simulink library "PC_Simulator_Lib"  (Simulink 8.2)
settings: Solver=ode45  StartTime=0.0  StopTime=10.0  RelTol=1e-3
values from neighbouring files (symbols this model uses):
  data = [r1 r2 r3 r4 L1 L2 L3 L4]    [strasse_Bedatung_HNI_ITI.m]
  distSameLane = 60    [InitialisationsEnv.m]
  eng_speed = [0 60 120 180 240 300 360 420 480 540 600 660 ... (101 elements, 1x101)]    [engine_table.mat]    (also in motor_parameter_calc.m = omega)
  Heading_init = 0    [Start.m]
  inertiaLateral = 25*(radiusWheel)^2    (= 4.129024)    [Start.m]
  laneWidth = 3.6    [InitialisationsEnv.m]    (also in strasse_Bedatung_HNI_ITI.m)
  omega_engine = [0.000000 150.000000 500.000000 1000.000000 1500.000000 2000.000000 2500.000000 3000.000000 3500.000000 4000.000000 4500.000000 5000.000000 5500.000000 6000.000000]    [friction_tables.m]
  omega_max = 6000    [engine_table.mat]    (also in motor_parameter_calc.m)
  omega_wheel = [0 20 40 60 80 100 122 143.7 164]    [friction_tables.m]
  para_Fellow_8_Points = ADAS.Fellow_8_Points    [ADAS_parameters.m]
  position_start_x = [x1 x2 x3 x4 x5 x6 x7]    [strasse_Bedatung_HNI_ITI.m]
  position_start_y = [y1 y2 y3 y4 y5 y6 y7]    [strasse_Bedatung_HNI_ITI.m]
  rad3rdLine = 57.2    [InitialisationsEnv.m]    (also in strasse_Bedatung_HNI_ITI.m)
  radiusWheel = 16*2.54/100    (= 0.4064)    [Start.m]
  s_values = [S1 S2 S3 S4 S5 S6 S7]    [strasse_Bedatung_HNI_ITI.m]
  segmentLimits = [segment1EndThirdLine                   segment2EndThirdLine                   segment3EndThirdLine                   segment4EndThirdLine                   segment5EndThirdLine                   segment6EndThirdLine                   segment7EndThirdLine                   segment8EndThirdLine                   ]    [InitialisationsEnv.m]    (also in strasse_Bedatung_HNI_ITI.m)
  setPosT = [-1.8 -5.4 -1.8 -5.4 -1.8 -5.4 -1.8 -5.4 -1.8 -5.4]    [InitialisationsEnv.m]
  torque = [297.089227105 300.997600937 304.800343044 308.497453426 312.088932082 315.574779014 318.95499422 322.229577701 325.398529457 328.461849487 331.419537793 334.271594373 ... (101 elements, 1x101)]    [engine_table.mat]    (also in motor_parameter_calc.m = g)
  Torque_lost = [0.000000 -8.777780 -15.000000 -26.800000 -29.600000 -32.700000 -35.900000 -39.300000 -42.800000 -46.500000 -50.300000 -54.300000 -58.500000 -62.800000 ]*0.6    [friction_tables.m]
  Torque_lost_wheel = [0.8 0.8 0.75 0.7 0.4 0.3 0.2 0.07 0.07]*0.2    [friction_tables.m]
  X_init = 0    [Start.m]
  Y_init = 1.8    [Start.m]
  Z_init = 0    [Start.m]
undefined symbols (not defined in the file or in its folder): Acc_Pedal, ADAS, Brake_Pedal, Joystick, Newton, Para, Raphson, Standard_Devices, Steering_Wheel_Angle, UDP_Protocol
libraries: simulink x43, rtwinlib x7, dspnetwork x2, simulink_extras x1, vrlib x1
(part 11 of 13)

== system PC_Simulator_Lib/Vehicle dynamics/Vertical_Dyn./suspention_System/Rear_Right_Suspention/vertical_dynamics_tire ==
  note: U
  note: F0
  note: z1
  Force_Suspention : Inport
  Vertical_Displacement_Z0_Road : Inport  Port=2
  intial_force_form_mass : Inport  Port=3
  1/Mu : Gain  Gain=1/Para.VD.wheel_Mass.v
  Add1 : Sum  Inputs=++-
  Add2 : Sum  Inputs=+-
  Gain : Gain  Gain=Para.VD.Tire_Stifness.v
  Gain2 : Gain  Gain=Para.VD.Tire_Damping_Constant.v
  Integrator : Integrator
  Integrator1 : Integrator
  Relational Operator : RelationalOperator  Operator=>  OutDataTypeStr=boolean  ZeroCross=off
  Saturation : Saturate  UpperLimit=Para.VD.Tire_intial_length.v-Para.VD.Tire_Lower_limit.v  LowerLimit=Para.VD.Tire_intial_length.v-Para.VD.Tire_Upper_limit.v
  Subtract2 : Sum  Inputs=+-
  Subtract3 : Sum  Inputs=+-
  Sum : Sum  Inputs=|++
  Switch : Switch
  Transfer Fcn : TransferFcn  Numerator=[1 0]  Denominator=[0.001 1]
  Transfer Fcn1 : TransferFcn  Numerator=[1 0]  Denominator=[0.001 1]
  Vertical_Displacement_Z1_Wheel : Outport
  Vertical_Velocity_Z1_Wheel : Outport  Port=2
  wires:
  Transfer Fcn1/1 -> Vertical_Velocity_Z1_Wheel/1
  Add1/1 -> 1/Mu/1
  1/Mu/1 -> Integrator/1
  Integrator/1 -> Integrator1/1, Subtract3/2
  Integrator1/1 -> Subtract2/2, Switch/3
  Subtract3/1 -> Gain2/1
  Gain2/1 -> Add1/2
  Saturation/1 -> Gain/1, Relational Operator/2, Add2/2
  Subtract2/1 -> Saturation/1, Relational Operator/1
  Transfer Fcn/1 -> Subtract3/1
  Vertical_Displacement_Z0_Road/1 -> Add2/1, Subtract2/1, Transfer Fcn/1
  Force_Suspention/1 -> Add1/3
  Gain/1 -> Sum/2
  Sum/1 -> Add1/1
  intial_force_form_mass/1 -> Sum/1
  Add2/1 -> Switch/1
  Relational Operator/1 -> Switch/2
  Switch/1 -> Transfer Fcn1/1, Vertical_Displacement_Z1_Wheel/1

== system PC_Simulator_Lib/Vehicle dynamics/Vertical_Dyn./suspention_System/Rear_left_Suspention/vertical_dynamics_tire ==
  note: U
  note: F0
  note: z1
  Force_Suspention : Inport
  Vertical_Displacement_Z0_Road : Inport  Port=2
  intial_force_form_mass : Inport  Port=3
  1/Mu : Gain  Gain=1/Para.VD.wheel_Mass.v
  Add1 : Sum  Inputs=++-
  Add2 : Sum  Inputs=+-
  Gain : Gain  Gain=Para.VD.Tire_Stifness.v
  Gain2 : Gain  Gain=Para.VD.Tire_Damping_Constant.v
  Integrator : Integrator
  Integrator1 : Integrator
  Relational Operator : RelationalOperator  Operator=>  OutDataTypeStr=boolean  ZeroCross=off
  Saturation : Saturate  UpperLimit=Para.VD.Tire_intial_length.v-Para.VD.Tire_Lower_limit.v  LowerLimit=Para.VD.Tire_intial_length.v-Para.VD.Tire_Upper_limit.v
  Subtract2 : Sum  Inputs=+-
  Subtract3 : Sum  Inputs=+-
  Sum : Sum  Inputs=|++
  Switch : Switch
  Transfer Fcn : TransferFcn  Numerator=[1 0]  Denominator=[0.001 1]
  Transfer Fcn1 : TransferFcn  Numerator=[1 0]  Denominator=[0.001 1]
  Vertical_Displacement_Z1_Wheel : Outport
  Vertical_Velocity_Z1_Wheel : Outport  Port=2
  wires:
  Transfer Fcn1/1 -> Vertical_Velocity_Z1_Wheel/1
  Add1/1 -> 1/Mu/1
  1/Mu/1 -> Integrator/1
  Integrator/1 -> Integrator1/1, Subtract3/2
  Integrator1/1 -> Subtract2/2, Switch/3
  Subtract3/1 -> Gain2/1
  Gain2/1 -> Add1/2
  Saturation/1 -> Gain/1, Relational Operator/2, Add2/2
  Subtract2/1 -> Saturation/1, Relational Operator/1
  Transfer Fcn/1 -> Subtract3/1
  Vertical_Displacement_Z0_Road/1 -> Add2/1, Subtract2/1, Transfer Fcn/1
  Force_Suspention/1 -> Add1/3
  Gain/1 -> Sum/2
  Sum/1 -> Add1/1
  intial_force_form_mass/1 -> Sum/1
  Add2/1 -> Switch/1
  Relational Operator/1 -> Switch/2
  Switch/1 -> Transfer Fcn1/1, Vertical_Displacement_Z1_Wheel/1

== system PC_Simulator_Lib/Vehicle dynamics/Vertical_Dyn./suspention_System/front_left_Suspention/vertical_dynamics_tire ==
  note: U
  note: F0
  note: z1
  Force_Suspention : Inport
  Vertical_Displacement_Z0_Road : Inport  Port=2
  intial_force_form_mass : Inport  Port=3
  1/Mu : Gain  Gain=1/Para.VD.wheel_Mass.v
  Add1 : Sum  Inputs=++-
  Add2 : Sum  Inputs=+-
  Gain : Gain  Gain=Para.VD.Tire_Stifness.v
  Gain2 : Gain  Gain=Para.VD.Tire_Damping_Constant.v
  Integrator : Integrator
  Integrator1 : Integrator
  Relational Operator : RelationalOperator  Operator=>  OutDataTypeStr=boolean  ZeroCross=off
  Saturation : Saturate  UpperLimit=Para.VD.Tire_intial_length.v-Para.VD.Tire_Lower_limit.v  LowerLimit=Para.VD.Tire_intial_length.v-Para.VD.Tire_Upper_limit.v
  Subtract2 : Sum  Inputs=+-
  Subtract3 : Sum  Inputs=+-
  Sum : Sum  Inputs=|++
  Switch : Switch
  Transfer Fcn : TransferFcn  Numerator=[1 0]  Denominator=[0.001 1]
  Transfer Fcn1 : TransferFcn  Numerator=[1 0]  Denominator=[0.001 1]
  Vertical_Displacement_Z1_Wheel : Outport
  Vertical_Velocity_Z1_Wheel : Outport  Port=2
  wires:
  Transfer Fcn1/1 -> Vertical_Velocity_Z1_Wheel/1
  Add1/1 -> 1/Mu/1
  1/Mu/1 -> Integrator/1
  Integrator/1 -> Integrator1/1, Subtract3/2
  Integrator1/1 -> Subtract2/2, Switch/3
  Subtract3/1 -> Gain2/1
  Gain2/1 -> Add1/2
  Saturation/1 -> Gain/1, Relational Operator/2, Add2/2
  Subtract2/1 -> Saturation/1, Relational Operator/1
  Transfer Fcn/1 -> Subtract3/1
  Vertical_Displacement_Z0_Road/1 -> Add2/1, Subtract2/1, Transfer Fcn/1
  Force_Suspention/1 -> Add1/3
  Gain/1 -> Sum/2
  Sum/1 -> Add1/1
  intial_force_form_mass/1 -> Sum/1
  Add2/1 -> Switch/1
  Relational Operator/1 -> Switch/2
  Switch/1 -> Transfer Fcn1/1, Vertical_Displacement_Z1_Wheel/1

== system PC_Simulator_Lib/Vehicle dynamics/Vertical_Dyn./suspention_System/front_right_Suspention/vertical_dynamics_tire ==
  note: U
  note: F0
  note: z1
  Force_Suspention : Inport
  Vertical_Displacement_Z0_Road : Inport  Port=2
  intial_force_form_mass : Inport  Port=3
  1/Mu : Gain  Gain=1/Para.VD.wheel_Mass.v
  Add1 : Sum  Inputs=++-
  Add2 : Sum  Inputs=+-
  Gain : Gain  Gain=Para.VD.Tire_Stifness.v
  Gain2 : Gain  Gain=Para.VD.Tire_Damping_Constant.v
  Integrator : Integrator
  Integrator1 : Integrator
  Relational Operator : RelationalOperator  Operator=>  OutDataTypeStr=boolean  ZeroCross=off
  Saturation : Saturate  UpperLimit=Para.VD.Tire_intial_length.v-Para.VD.Tire_Lower_limit.v  LowerLimit=Para.VD.Tire_intial_length.v-Para.VD.Tire_Upper_limit.v
  Subtract2 : Sum  Inputs=+-
  Subtract3 : Sum  Inputs=+-
  Sum : Sum  Inputs=|++
  Switch : Switch
  Transfer Fcn : TransferFcn  Numerator=[1 0]  Denominator=[0.001 1]
  Transfer Fcn1 : TransferFcn  Numerator=[1 0]  Denominator=[0.001 1]
  Vertical_Displacement_Z1_Wheel : Outport
  Vertical_Velocity_Z1_Wheel : Outport  Port=2
  wires:
  Transfer Fcn1/1 -> Vertical_Velocity_Z1_Wheel/1
  Add1/1 -> 1/Mu/1
  1/Mu/1 -> Integrator/1
  Integrator/1 -> Integrator1/1, Subtract3/2
  Integrator1/1 -> Subtract2/2, Switch/3
  Subtract3/1 -> Gain2/1
  Gain2/1 -> Add1/2
  Saturation/1 -> Gain/1, Relational Operator/2, Add2/2
  Subtract2/1 -> Saturation/1, Relational Operator/1
  Transfer Fcn/1 -> Subtract3/1
  Vertical_Displacement_Z0_Road/1 -> Add2/1, Subtract2/1, Transfer Fcn/1
  Force_Suspention/1 -> Add1/3
  Gain/1 -> Sum/2
  Sum/1 -> Add1/1
  intial_force_form_mass/1 -> Sum/1
  Add2/1 -> Switch/1
  Relational Operator/1 -> Switch/2
  Switch/1 -> Transfer Fcn1/1, Vertical_Displacement_Z1_Wheel/1

== system PC_Simulator_Lib/ADAS/Decision_Making_ADAS/Trajectory_calculatin_and_distance_control_and output_maping/Calculate_Desired_Trajectory/applying_Desired_T_Gradually/Triggered Subsystem ==
  In1 : Inport
  Trigger : TriggerPort  TriggerType=either
  Out1 : Outport
  wires:
  In1/1 -> Out1/1

== system PC_Simulator_Lib/ADAS/Decision_Making_ADAS/Trajectory_calculatin_and_distance_control_and output_maping/Distance_Control/Distance controller/Control_law ==
  Distance_desired[m] : Inport
  Distance_acctual[m] : Inport  Port=2
  V_realtive[m|s] : Inport  Port=3
  V_Vehicle[m|s] : Inport  Port=4
  V_Desired_max[m|s] : Inport  Port=5
  V_Desired_min[m|s] : Inport  Port=6
  Enable : EnablePort  StatesWhenEnabling=reset
  Add : Sum  Inputs=+++
  Add1 : Sum
  Add2 : Sum
  Ground : Ground
  Integrator : Integrator
  Kb : Gain  Gain=0.02
  Ki : Gain  Gain=0.001
  Kp : Gain  Gain=0.2
  Saturation Dynamic : simulink/Discontinuities/Saturation Dynamic  OutMin=[]  OutMax=[]  OutDataTypeStr=Inherit: Same as second input  OutDataType=fixdt(1, 16)  OutScaling=2^-10  DoSatur=off
  Subtract1 : Sum  Inputs=-+
  Subtract2 : Sum  Inputs=-+
  Terminator : Terminator
  V_Desired_Following[m|s] : Outport
  wires:
  Distance_desired[m]/1 -> Subtract1/1
  Distance_acctual[m]/1 -> Subtract1/2
  Subtract1/1 -> Kp/1, Ki/1
  Integrator/1 -> Terminator/1
  Kp/1 -> Add/2
  Add1/1 -> Integrator/1
  Ki/1 -> Add1/1
  Kb/1 -> Add1/2
  Saturation Dynamic/1 -> V_Desired_Following[m|s]/1, Subtract2/2
  V_Desired_max[m|s]/1 -> Saturation Dynamic/1
  V_Desired_min[m|s]/1 -> Saturation Dynamic/3
  Add/1 -> Saturation Dynamic/2, Subtract2/1
  V_Vehicle[m|s]/1 -> Add2/2
  V_realtive[m|s]/1 -> Add2/1
  Add2/1 -> Add/1
  Subtract2/1 -> Kb/1
  Ground/1 -> Add/3

== system PC_Simulator_Lib/ADAS/Decision_Making_ADAS/Trajectory_calculatin_and_distance_control_and output_maping/Distance_Control/Distance controller/Enable_Distance_Controller ==
  S_Start_Braking[m] : Inport
  Distance_2_Felow_Vehicle[m] : Inport  Port=2
  V_realtive[m|s] : Inport  Port=3
  V_Vehicle[m|s] : Inport  Port=4
  V_User_Set_Speed[m|s] : Inport  Port=5
  Add2 : Sum
  Gain : Gain  Gain=1.2
  Logical Operator : Logic  AllPortsSameDT=off  OutDataTypeStr=boolean
  Relational Operator : RelationalOperator  Operator=>  OutDataTypeStr=boolean
  Relational Operator1 : RelationalOperator  Operator=<  OutDataTypeStr=boolean
  Relational Operator2 : RelationalOperator  Operator=>  OutDataTypeStr=boolean
  S-R Flip-Flop : simulink_extras/Flip Flops/S-R Flip-Flop  initial_condition=0
  Terminator : Terminator
  Enable_Distance_Controller : Outport
  wires:
  Distance_2_Felow_Vehicle[m]/1 -> Relational Operator1/2, Relational Operator/2
  S_Start_Braking[m]/1 -> Gain/1, Relational Operator/1
  Relational Operator/1 -> S-R Flip-Flop/1
  S-R Flip-Flop/2 -> Terminator/1
  Relational Operator1/1 -> Logical Operator/1
  V_realtive[m|s]/1 -> Add2/1
  V_Vehicle[m|s]/1 -> Add2/2
  Add2/1 -> Relational Operator2/1
  V_User_Set_Speed[m|s]/1 -> Relational Operator2/2
  Logical Operator/1 -> S-R Flip-Flop/2
  Relational Operator2/1 -> Logical Operator/2
  S-R Flip-Flop/1 -> Enable_Distance_Controller/1
  Gain/1 -> Relational Operator1/1

== system PC_Simulator_Lib/ADAS/Execution_ADAS/Longitudinal_Controller/Acceleration_Control/Tractive_Force_Required_determination/Force_of_Aerodynamics ==
  Vx_CoG[m|s] : Inport
  Gain : Gain  Gain=Para.VD.Air_Risistance_Coefficient.v
  Math Function : Math  Operator=square  SaturateOnIntegerOverflow=on
  Product2 : Product  RndMeth=Zero
  Sign : Signum
  Force_of_aerodynamics_in_X : Outport
  wires:
  Vx_CoG[m|s]/1 -> Math Function/1, Sign/1
  Sign/1 -> Product2/2
  Gain/1 -> Product2/1
  Product2/1 -> Force_of_aerodynamics_in_X/1
  Math Function/1 -> Gain/1

== system PC_Simulator_Lib/ADAS/Execution_ADAS/Longitudinal_Controller/Acceleration_Control/Tractive_Force_Required_determination/Friction_FL ==
  omega_radPs : Inport
  Lookup Table : Lookup_n-D  NumberOfTableDimensions=1  BreakpointsForDimension1=omega_wheel  BeginIndexSearchUsingPreviousIndexResult=on  Table=Torque_lost_wheel  InputSameDT=on
  Product : Product  RndMeth=Zero
  Torque_friction : Outport
  wires:
  omega_radPs/1 -> Product/2, Lookup Table/1
  Product/1 -> Torque_friction/1
  Lookup Table/1 -> Product/1

== system PC_Simulator_Lib/ADAS/Execution_ADAS/Longitudinal_Controller/Acceleration_Control/Tractive_Force_Required_determination/Friction_FR ==
  omega_radPs : Inport
  Lookup Table : Lookup_n-D  NumberOfTableDimensions=1  BreakpointsForDimension1=omega_wheel  BeginIndexSearchUsingPreviousIndexResult=on  Table=Torque_lost_wheel  InputSameDT=on
  Product : Product  RndMeth=Zero
  Torque_friction : Outport
  wires:
  Lookup Table/1 -> Product/1
  Product/1 -> Torque_friction/1
  omega_radPs/1 -> Lookup Table/1, Product/2

== system PC_Simulator_Lib/ADAS/Execution_ADAS/Longitudinal_Controller/Acceleration_Control/Tractive_Force_Required_determination/Friction_RL ==
  omega_radPs : Inport
  Lookup Table : Lookup_n-D  NumberOfTableDimensions=1  BreakpointsForDimension1=omega_wheel  BeginIndexSearchUsingPreviousIndexResult=on  Table=Torque_lost_wheel  InputSameDT=on
  Product : Product  RndMeth=Zero
  Torque_friction : Outport
  wires:
  omega_radPs/1 -> Product/2, Lookup Table/1
  Product/1 -> Torque_friction/1
  Lookup Table/1 -> Product/1

== system PC_Simulator_Lib/ADAS/Execution_ADAS/Longitudinal_Controller/Acceleration_Control/Tractive_Force_Required_determination/Friction_RR ==
  omega_radPs : Inport
  Lookup Table : Lookup_n-D  NumberOfTableDimensions=1  BreakpointsForDimension1=omega_wheel  BeginIndexSearchUsingPreviousIndexResult=on  Table=Torque_lost_wheel  InputSameDT=on
  Product : Product  RndMeth=Zero
  Torque_friction : Outport
  wires:
  Lookup Table/1 -> Product/1
  Product/1 -> Torque_friction/1
  omega_radPs/1 -> Lookup Table/1, Product/2

== system PC_Simulator_Lib/ADAS/Sensors_ADAS/Front_Long_Range_Radar_Sensor/First_STage_Coordinate_Transformation/Radar_Triangles_Transformation_From_Local2Global/Pitch_angle_offset ==
  Constant : Constant  Value=0.02
  Constant1 : Constant  Value=7*pi/180
  Digital Clock : DigitalClock  SampleTime=0.001
  Gain : Gain  Gain=1000
  Gain1 : Gain  Gain=atan(1/250)*3
  Math Function : Math  Operator=rem  SaturateOnIntegerOverflow=on
  Subtract : Sum  Inputs=+-
  Delta_pitch_angle[rad] : Outport
  Round_done[bool] : Outport  Port=2
  wires:
  Digital Clock/1 -> Math Function/1
  Gain1/1 -> Subtract/1
  Constant/1 -> Math Function/2
  Gain/1 -> Gain1/1, Round_done[bool]/1
  Math Function/1 -> Gain/1
  Subtract/1 -> Delta_pitch_angle[rad]/1
  Constant1/1 -> Subtract/2

== system PC_Simulator_Lib/ADAS/Sensors_ADAS/Front_Long_Range_Radar_Sensor/First_STage_Coordinate_Transformation/Radar_Triangles_Transformation_From_Local2Global/Subsystem ==
  Transformation_Local2Global : Inport
  Position_of_Origine_Local_coord[m] : Inport  Port=2
  Positon_Local[m] : Inport  Port=3
  Add1 : Sum
  Product1 : Product  Multiplication=Matrix(*)
  Position_Global[m] : Outport
  wires:
  Positon_Local[m]/1 -> Product1/2
  Transformation_Local2Global/1 -> Product1/1
  Position_of_Origine_Local_coord[m]/1 -> Add1/2
  Add1/1 -> Position_Global[m]/1
  Product1/1 -> Add1/1

== system PC_Simulator_Lib/ADAS/Sensors_ADAS/Front_Long_Range_Radar_Sensor/First_STage_Coordinate_Transformation/Radar_Triangles_Transformation_From_Local2Global/Subsystem1 ==
  Transformation_Local2Global : Inport
  Position_of_Origine_Local_coord[m] : Inport  Port=2
  Positon_Local[m] : Inport  Port=3
  Add1 : Sum
  Product1 : Product  Multiplication=Matrix(*)
  Position_Global[m] : Outport
  wires:
  Product1/1 -> Add1/1
  Add1/1 -> Position_Global[m]/1
  Position_of_Origine_Local_coord[m]/1 -> Add1/2
  Transformation_Local2Global/1 -> Product1/1
  Positon_Local[m]/1 -> Product1/2

== system PC_Simulator_Lib/ADAS/Sensors_ADAS/Front_Long_Range_Radar_Sensor/First_STage_Coordinate_Transformation/Radar_Triangles_Transformation_From_Local2Global/Subsystem2 ==
  Transformation_Local2Global : Inport
  Position_of_Origine_Local_coord[m] : Inport  Port=2
  Positon_Local[m] : Inport  Port=3
  Add1 : Sum
  Product1 : Product  Multiplication=Matrix(*)
  Position_Global[m] : Outport
  wires:
  Positon_Local[m]/1 -> Product1/2
  Transformation_Local2Global/1 -> Product1/1
  Position_of_Origine_Local_coord[m]/1 -> Add1/2
  Add1/1 -> Position_Global[m]/1
  Product1/1 -> Add1/1

== system PC_Simulator_Lib/ADAS/Sensors_ADAS/Front_Long_Range_Radar_Sensor/First_STage_Coordinate_Transformation/Radar_Triangles_Transformation_From_Local2Global/Subsystem3 ==
  Transformation_Local2Global : Inport
  Position_of_Origine_Local_coord[m] : Inport  Port=2
  Positon_Local[m] : Inport  Port=3
  Add1 : Sum
  Product1 : Product  Multiplication=Matrix(*)
  Position_Global[m] : Outport
  wires:
  Product1/1 -> Add1/1
  Add1/1 -> Position_Global[m]/1
  Position_of_Origine_Local_coord[m]/1 -> Add1/2
  Transformation_Local2Global/1 -> Product1/1
  Positon_Local[m]/1 -> Product1/2

== system PC_Simulator_Lib/ADAS/Sensors_ADAS/Front_Long_Range_Radar_Sensor/First_STage_Coordinate_Transformation/Radar_Triangles_Transformation_From_Local2Global/Subsystem4 ==
  Transformation_Local2Global : Inport
  Position_of_Origine_Local_coord[m] : Inport  Port=2
  Positon_Local[m] : Inport  Port=3
  Add1 : Sum
  Product1 : Product  Multiplication=Matrix(*)
  Position_Global[m] : Outport
  wires:
  Positon_Local[m]/1 -> Product1/2
  Transformation_Local2Global/1 -> Product1/1
  Position_of_Origine_Local_coord[m]/1 -> Add1/2
  Add1/1 -> Position_Global[m]/1
  Product1/1 -> Add1/1

== system PC_Simulator_Lib/ADAS/Sensors_ADAS/Front_Long_Range_Radar_Sensor/First_STage_Coordinate_Transformation/Radar_Triangles_Transformation_From_Local2Global/Subsystem5 ==
  Transformation_Local2Global : Inport
  Position_of_Origine_Local_coord[m] : Inport  Port=2
  Positon_Local[m] : Inport  Port=3
  Add1 : Sum
  Product1 : Product  Multiplication=Matrix(*)
  Position_Global[m] : Outport
  wires:
  Product1/1 -> Add1/1
  Add1/1 -> Position_Global[m]/1
  Position_of_Origine_Local_coord[m]/1 -> Add1/2
  Transformation_Local2Global/1 -> Product1/1
  Positon_Local[m]/1 -> Product1/2

== system PC_Simulator_Lib/ADAS/Sensors_ADAS/Front_Long_Range_Radar_Sensor/First_STage_Coordinate_Transformation/Radar_Triangles_Transformation_From_Local2Global/Subsystem6 ==
  Transformation_Local2Global : Inport
  Position_of_Origine_Local_coord[m] : Inport  Port=2
  Positon_Local[m] : Inport  Port=3
  Add1 : Sum
  Product1 : Product  Multiplication=Matrix(*)
  Position_Global[m] : Outport
  wires:
  Positon_Local[m]/1 -> Product1/2
  Transformation_Local2Global/1 -> Product1/1
  Position_of_Origine_Local_coord[m]/1 -> Add1/2
  Add1/1 -> Position_Global[m]/1
  Product1/1 -> Add1/1

== system PC_Simulator_Lib/ADAS/Sensors_ADAS/Front_Long_Range_Radar_Sensor/First_STage_Coordinate_Transformation/Radar_Triangles_Transformation_From_Local2Global/Subsystem7 ==
  Transformation_Local2Global : Inport
  Position_of_Origine_Local_coord[m] : Inport  Port=2
  Positon_Local[m] : Inport  Port=3
  Add1 : Sum
  Product1 : Product  Multiplication=Matrix(*)
  Position_Global[m] : Outport
  wires:
  Product1/1 -> Add1/1
  Add1/1 -> Position_Global[m]/1
  Position_of_Origine_Local_coord[m]/1 -> Add1/2
  Transformation_Local2Global/1 -> Product1/1
  Positon_Local[m]/1 -> Product1/2

== system PC_Simulator_Lib/ADAS/Sensors_ADAS/Front_Mid_Range_Radar_Sensor/First_STage_Coordinate_Transformation/Radar_Triangles_Transformation_From_Local2Global/Pitch_angle_offset ==
  Constant : Constant  Value=0.02
  Constant1 : Constant  Value=7*pi/180
  Digital Clock : DigitalClock  SampleTime=0.001
  Gain : Gain  Gain=1000
  Gain1 : Gain  Gain=atan(1/250)*3
  Math Function : Math  Operator=rem  SaturateOnIntegerOverflow=on
  Subtract : Sum  Inputs=+-
  Delta_pitch_angle[rad] : Outport
  Round_done[bool] : Outport  Port=2
  wires:
  Digital Clock/1 -> Math Function/1
  Gain1/1 -> Subtract/1
  Constant/1 -> Math Function/2
  Gain/1 -> Gain1/1, Round_done[bool]/1
  Math Function/1 -> Gain/1
  Subtract/1 -> Delta_pitch_angle[rad]/1
  Constant1/1 -> Subtract/2

== system PC_Simulator_Lib/ADAS/Sensors_ADAS/Front_Mid_Range_Radar_Sensor/First_STage_Coordinate_Transformation/Radar_Triangles_Transformation_From_Local2Global/Subsystem ==
  Transformation_Local2Global : Inport
  Position_of_Origine_Local_coord[m] : Inport  Port=2
  Positon_Local[m] : Inport  Port=3
  Add1 : Sum
  Product1 : Product  Multiplication=Matrix(*)
  Position_Global[m] : Outport
  wires:
  Positon_Local[m]/1 -> Product1/2
  Transformation_Local2Global/1 -> Product1/1
  Position_of_Origine_Local_coord[m]/1 -> Add1/2
  Add1/1 -> Position_Global[m]/1
  Product1/1 -> Add1/1

== system PC_Simulator_Lib/ADAS/Sensors_ADAS/Front_Mid_Range_Radar_Sensor/First_STage_Coordinate_Transformation/Radar_Triangles_Transformation_From_Local2Global/Subsystem1 ==
  Transformation_Local2Global : Inport
  Position_of_Origine_Local_coord[m] : Inport  Port=2
  Positon_Local[m] : Inport  Port=3
  Add1 : Sum
  Product1 : Product  Multiplication=Matrix(*)
  Position_Global[m] : Outport
  wires:
  Product1/1 -> Add1/1
  Add1/1 -> Position_Global[m]/1
  Position_of_Origine_Local_coord[m]/1 -> Add1/2
  Transformation_Local2Global/1 -> Product1/1
  Positon_Local[m]/1 -> Product1/2

== system PC_Simulator_Lib/ADAS/Sensors_ADAS/Front_Mid_Range_Radar_Sensor/First_STage_Coordinate_Transformation/Radar_Triangles_Transformation_From_Local2Global/Subsystem2 ==
  Transformation_Local2Global : Inport
  Position_of_Origine_Local_coord[m] : Inport  Port=2
  Positon_Local[m] : Inport  Port=3
  Add1 : Sum
  Product1 : Product  Multiplication=Matrix(*)
  Position_Global[m] : Outport
  wires:
  Positon_Local[m]/1 -> Product1/2
  Transformation_Local2Global/1 -> Product1/1
  Position_of_Origine_Local_coord[m]/1 -> Add1/2
  Add1/1 -> Position_Global[m]/1
  Product1/1 -> Add1/1

== system PC_Simulator_Lib/ADAS/Sensors_ADAS/Front_Mid_Range_Radar_Sensor/First_STage_Coordinate_Transformation/Radar_Triangles_Transformation_From_Local2Global/Subsystem3 ==
  Transformation_Local2Global : Inport
  Position_of_Origine_Local_coord[m] : Inport  Port=2
  Positon_Local[m] : Inport  Port=3
  Add1 : Sum
  Product1 : Product  Multiplication=Matrix(*)
  Position_Global[m] : Outport
  wires:
  Product1/1 -> Add1/1
  Add1/1 -> Position_Global[m]/1
  Position_of_Origine_Local_coord[m]/1 -> Add1/2
  Transformation_Local2Global/1 -> Product1/1
  Positon_Local[m]/1 -> Product1/2

== system PC_Simulator_Lib/ADAS/Sensors_ADAS/Front_Mid_Range_Radar_Sensor/First_STage_Coordinate_Transformation/Radar_Triangles_Transformation_From_Local2Global/Subsystem4 ==
  Transformation_Local2Global : Inport
  Position_of_Origine_Local_coord[m] : Inport  Port=2
  Positon_Local[m] : Inport  Port=3
  Add1 : Sum
  Product1 : Product  Multiplication=Matrix(*)
  Position_Global[m] : Outport
  wires:
  Positon_Local[m]/1 -> Product1/2
  Transformation_Local2Global/1 -> Product1/1
  Position_of_Origine_Local_coord[m]/1 -> Add1/2
  Add1/1 -> Position_Global[m]/1
  Product1/1 -> Add1/1

== system PC_Simulator_Lib/ADAS/Sensors_ADAS/Front_Mid_Range_Radar_Sensor/First_STage_Coordinate_Transformation/Radar_Triangles_Transformation_From_Local2Global/Subsystem5 ==
  Transformation_Local2Global : Inport
  Position_of_Origine_Local_coord[m] : Inport  Port=2
  Positon_Local[m] : Inport  Port=3
  Add1 : Sum
  Product1 : Product  Multiplication=Matrix(*)
  Position_Global[m] : Outport
  wires:
  Product1/1 -> Add1/1
  Add1/1 -> Position_Global[m]/1
  Position_of_Origine_Local_coord[m]/1 -> Add1/2
  Transformation_Local2Global/1 -> Product1/1
  Positon_Local[m]/1 -> Product1/2

== system PC_Simulator_Lib/ADAS/Sensors_ADAS/Front_Mid_Range_Radar_Sensor/First_STage_Coordinate_Transformation/Radar_Triangles_Transformation_From_Local2Global/Subsystem6 ==
  Transformation_Local2Global : Inport
  Position_of_Origine_Local_coord[m] : Inport  Port=2
  Positon_Local[m] : Inport  Port=3
  Add1 : Sum
  Product1 : Product  Multiplication=Matrix(*)
  Position_Global[m] : Outport
  wires:
  Positon_Local[m]/1 -> Product1/2
  Transformation_Local2Global/1 -> Product1/1
  Position_of_Origine_Local_coord[m]/1 -> Add1/2
  Add1/1 -> Position_Global[m]/1
  Product1/1 -> Add1/1

== system PC_Simulator_Lib/ADAS/Sensors_ADAS/Front_Mid_Range_Radar_Sensor/First_STage_Coordinate_Transformation/Radar_Triangles_Transformation_From_Local2Global/Subsystem7 ==
  Transformation_Local2Global : Inport
  Position_of_Origine_Local_coord[m] : Inport  Port=2
  Positon_Local[m] : Inport  Port=3
  Add1 : Sum
  Product1 : Product  Multiplication=Matrix(*)
  Position_Global[m] : Outport
  wires:
  Product1/1 -> Add1/1
  Add1/1 -> Position_Global[m]/1
  Position_of_Origine_Local_coord[m]/1 -> Add1/2
  Transformation_Local2Global/1 -> Product1/1
  Positon_Local[m]/1 -> Product1/2

== system PC_Simulator_Lib/ADAS/Sensors_ADAS/Input_Maping/Fellows/Subsystem2/Subsystem1 ==
  In1 : Inport
  Constant9 : Constant  Value=Z_init
  Sum : Sum  Inputs=|++
  Out1 : Outport
  wires:
  Sum/1 -> Out1/1
  Constant9/1 -> Sum/2
  In1/1 -> Sum/1

== system PC_Simulator_Lib/ADAS/Sensors_ADAS/Input_Maping/Fellows/Subsystem2/Subsystem10 ==
  In1 : Inport
  Constant9 : Constant  Value=Z_init
  Sum : Sum  Inputs=|++
  Out1 : Outport
  wires:
  Sum/1 -> Out1/1
  Constant9/1 -> Sum/2
  In1/1 -> Sum/1

== system PC_Simulator_Lib/ADAS/Sensors_ADAS/Input_Maping/Fellows/Subsystem2/Subsystem2 ==
  In1 : Inport
  Constant9 : Constant  Value=Z_init
  Sum : Sum  Inputs=|++
  Out1 : Outport
  wires:
  In1/1 -> Sum/1
  Constant9/1 -> Sum/2
  Sum/1 -> Out1/1

== system PC_Simulator_Lib/ADAS/Sensors_ADAS/Input_Maping/Fellows/Subsystem2/Subsystem3 ==
  In1 : Inport
  Constant9 : Constant  Value=Z_init
  Sum : Sum  Inputs=|++
  Out1 : Outport
  wires:
  Sum/1 -> Out1/1
  Constant9/1 -> Sum/2
  In1/1 -> Sum/1

== system PC_Simulator_Lib/ADAS/Sensors_ADAS/Input_Maping/Fellows/Subsystem2/Subsystem4 ==
  In1 : Inport
  Constant9 : Constant  Value=Z_init
  Sum : Sum  Inputs=|++
  Out1 : Outport
  wires:
  In1/1 -> Sum/1
  Constant9/1 -> Sum/2
  Sum/1 -> Out1/1

== system PC_Simulator_Lib/ADAS/Sensors_ADAS/Input_Maping/Fellows/Subsystem2/Subsystem5 ==
  In1 : Inport
  Constant9 : Constant  Value=Z_init
  Sum : Sum  Inputs=|++
  Out1 : Outport
  wires:
  Sum/1 -> Out1/1
  Constant9/1 -> Sum/2
  In1/1 -> Sum/1

== system PC_Simulator_Lib/ADAS/Sensors_ADAS/Input_Maping/Fellows/Subsystem2/Subsystem6 ==
  In1 : Inport
  Constant9 : Constant  Value=Z_init
  Sum : Sum  Inputs=|++
  Out1 : Outport
  wires:
  In1/1 -> Sum/1
  Constant9/1 -> Sum/2
  Sum/1 -> Out1/1

== system PC_Simulator_Lib/ADAS/Sensors_ADAS/Input_Maping/Fellows/Subsystem2/Subsystem7 ==
  In1 : Inport
  Constant9 : Constant  Value=Z_init
  Sum : Sum  Inputs=|++
  Out1 : Outport
  wires:
  Sum/1 -> Out1/1
  Constant9/1 -> Sum/2
  In1/1 -> Sum/1

== system PC_Simulator_Lib/ADAS/Sensors_ADAS/Input_Maping/Fellows/Subsystem2/Subsystem8 ==
  In1 : Inport
  Constant9 : Constant  Value=Z_init
  Sum : Sum  Inputs=|++
  Out1 : Outport
  wires:
  In1/1 -> Sum/1
  Constant9/1 -> Sum/2
  Sum/1 -> Out1/1

== system PC_Simulator_Lib/ADAS/Sensors_ADAS/Input_Maping/Fellows/Subsystem2/Subsystem9 ==
  In1 : Inport
  Constant9 : Constant  Value=Z_init
  Sum : Sum  Inputs=|++
  Out1 : Outport
  wires:
  In1/1 -> Sum/1
  Constant9/1 -> Sum/2
  Sum/1 -> Out1/1

== system PC_Simulator_Lib/Drive_Train/4_Wheels_drive_train_and_Brake/FL/Alpha_Kappa_Selector2/Dynamik Anteil2/Subsystem3 ==
  In1 : Inport
  Abs : Abs  SaturateOnIntegerOverflow=on
  In3_Switch : Constant
  Relational Operator : RelationalOperator
  Switch : Switch  Threshold=1  SaturateOnIntegerOverflow=on
  Out1 : Outport
  wires:
  In1/1 -> Switch/1, Abs/1
  Abs/1 -> Relational Operator/1
  In3_Switch/1 -> Relational Operator/2, Switch/3
  Relational Operator/1 -> Switch/2
  Switch/1 -> Out1/1

== system PC_Simulator_Lib/Drive_Train/4_Wheels_drive_train_and_Brake/FL/Alpha_Kappa_Selector2/alpha_calc/Slip_angle_Calculation_From_Vx_and_Vy1 ==
  Vx_CoG[m|s] : Inport
  Vy_CoG[m|s] : Inport  Port=2
  Add : Sum
  Add2 : Sum
  Compare To Constant1 : simulink/Logic and Bit Operations/Compare To Constant  relop=>=  const=1  OutDataTypeStr=boolean
  Constant1 : Constant  Value=eps
  Data Type Conversion : DataTypeConversion
  Divide : Product  Inputs=*/
  Gain : Gain  Gain=180/pi
  Math Function : Math  Operator=square  SaturateOnIntegerOverflow=on
  Math Function1 : Math  Operator=square  SaturateOnIntegerOverflow=on
  Product1 : Product  Inputs=3
  Sign : Signum
  Sqrt : Sqrt  AlgorithmType=Newton-Raphson  SaturateOnIntegerOverflow=on
  Trigonometric Function1 : Trigonometry  Operator=atan
  Unary Minus1 : UnaryMinus
  Slip_Angle[deg] : Outport
  wires:
  Gain/1 -> Slip_Angle[deg]/1
  Product1/1 -> Gain/1
  Data Type Conversion/1 -> Product1/2
  Compare To Constant1/1 -> Data Type Conversion/1
  Vy_CoG[m|s]/1 -> Math Function1/1, Divide/1
  Vx_CoG[m|s]/1 -> Sign/1, Math Function/1, Add2/1
  Math Function/1 -> Add/1
  Math Function1/1 -> Add/2
  Add/1 -> Sqrt/1
  Sqrt/1 -> Compare To Constant1/1
  Divide/1 -> Trigonometric Function1/1
  Add2/1 -> Divide/2
  Constant1/1 -> Add2/2
  Trigonometric Function1/1 -> Product1/1
  Sign/1 -> Unary Minus1/1
  Unary Minus1/1 -> Product1/3

== system PC_Simulator_Lib/Drive_Train/4_Wheels_drive_train_and_Brake/FL/Alpha_Kappa_Selector2/alpha_calc/front ==
  Vy : Inport
  Vx : Inport  Port=2
  steering_angle : Inport  Port=3
  Constant : Constant  Value=0.001
  Divide : Product  Inputs=*/
  Fcn : Fcn  Expr=atan(u)
  Gain : Gain  Gain=180/pi
  Relational Operator : RelationalOperator  OutDataTypeStr=boolean
  Subsystem1 : Subsystem
  Subtract : Sum  Inputs=+-
  Switch : Switch  Threshold=1
  alpha : Outport
  wires:
  Relational Operator/1 -> Switch/2
  Constant/1 -> Switch/3, Relational Operator/2
  steering_angle/1 -> Subtract/1
  Subtract/1 -> Gain/1
  Divide/1 -> Fcn/1
  Gain/1 -> alpha/1
  Fcn/1 -> Subtract/2
  Switch/1 -> Divide/2
  Vy/1 -> Subsystem1/1(In1)
  Vx/1 -> Relational Operator/1, Switch/1
  Subsystem1/1(Out1) -> Divide/1

== system PC_Simulator_Lib/Drive_Train/4_Wheels_drive_train_and_Brake/FR/Alpha_Kappa_Selector2/Dynamik Anteil2/Subsystem3 ==
  In1 : Inport
  Abs : Abs  SaturateOnIntegerOverflow=on
  In3_Switch : Constant
  Relational Operator : RelationalOperator
  Switch : Switch  Threshold=1  SaturateOnIntegerOverflow=on
  Out1 : Outport
  wires:
  In1/1 -> Switch/1, Abs/1
  Abs/1 -> Relational Operator/1
  In3_Switch/1 -> Relational Operator/2, Switch/3
  Relational Operator/1 -> Switch/2
  Switch/1 -> Out1/1

== system PC_Simulator_Lib/Drive_Train/4_Wheels_drive_train_and_Brake/FR/Alpha_Kappa_Selector2/alpha_calc/Slip_angle_Calculation_From_Vx_and_Vy1 ==
  Vx_CoG[m|s] : Inport
  Vy_CoG[m|s] : Inport  Port=2
  Add : Sum
  Add2 : Sum
  Compare To Constant1 : simulink/Logic and Bit Operations/Compare To Constant  relop=>=  const=1  OutDataTypeStr=boolean
  Constant1 : Constant  Value=eps
  Data Type Conversion : DataTypeConversion
  Divide : Product  Inputs=*/
  Gain : Gain  Gain=180/pi
  Math Function : Math  Operator=square  SaturateOnIntegerOverflow=on
  Math Function1 : Math  Operator=square  SaturateOnIntegerOverflow=on
  Product1 : Product  Inputs=3
  Sign : Signum
  Sqrt : Sqrt  AlgorithmType=Newton-Raphson  SaturateOnIntegerOverflow=on
  Trigonometric Function1 : Trigonometry  Operator=atan
  Unary Minus1 : UnaryMinus
  Slip_Angle[deg] : Outport
  wires:
  Gain/1 -> Slip_Angle[deg]/1
  Product1/1 -> Gain/1
  Data Type Conversion/1 -> Product1/2
  Compare To Constant1/1 -> Data Type Conversion/1
  Vy_CoG[m|s]/1 -> Math Function1/1, Divide/1
  Vx_CoG[m|s]/1 -> Sign/1, Math Function/1, Add2/1
  Math Function/1 -> Add/1
  Math Function1/1 -> Add/2
  Add/1 -> Sqrt/1
  Sqrt/1 -> Compare To Constant1/1
  Divide/1 -> Trigonometric Function1/1
  Add2/1 -> Divide/2
  Constant1/1 -> Add2/2
  Trigonometric Function1/1 -> Product1/1
  Sign/1 -> Unary Minus1/1
  Unary Minus1/1 -> Product1/3

== system PC_Simulator_Lib/Drive_Train/4_Wheels_drive_train_and_Brake/FR/Alpha_Kappa_Selector2/alpha_calc/front ==
  Vy : Inport
  Vx : Inport  Port=2
  steering_angle : Inport  Port=3
  Constant : Constant  Value=0.001
  Divide : Product  Inputs=*/
  Fcn : Fcn  Expr=atan(u)
  Gain : Gain  Gain=180/pi
  Relational Operator : RelationalOperator  OutDataTypeStr=boolean
  Subsystem1 : Subsystem
  Subtract : Sum  Inputs=+-
  Switch : Switch  Threshold=1
  alpha : Outport
  wires:
  Relational Operator/1 -> Switch/2
  Constant/1 -> Switch/3, Relational Operator/2
  steering_angle/1 -> Subtract/1
  Subtract/1 -> Gain/1
  Divide/1 -> Fcn/1
  Gain/1 -> alpha/1
  Fcn/1 -> Subtract/2
  Switch/1 -> Divide/2
  Vy/1 -> Subsystem1/1(In1)
  Vx/1 -> Relational Operator/1, Switch/1
  Subsystem1/1(Out1) -> Divide/1

== system PC_Simulator_Lib/Drive_Train/4_Wheels_drive_train_and_Brake/RL/Alpha_Kappa_Selector2/Dynamik Anteil2/Subsystem3 ==
  In1 : Inport
  Abs : Abs  SaturateOnIntegerOverflow=on
  In3_Switch : Constant
  Relational Operator : RelationalOperator
  Switch : Switch  Threshold=1  SaturateOnIntegerOverflow=on
  Out1 : Outport
  wires:
  In1/1 -> Switch/1, Abs/1
  Abs/1 -> Relational Operator/1
  In3_Switch/1 -> Relational Operator/2, Switch/3
  Relational Operator/1 -> Switch/2
  Switch/1 -> Out1/1

== system PC_Simulator_Lib/Drive_Train/4_Wheels_drive_train_and_Brake/RL/Alpha_Kappa_Selector2/alpha_calc/Slip_angle_Calculation_From_Vx_and_Vy1 ==
  Vx_CoG[m|s] : Inport
  Vy_CoG[m|s] : Inport  Port=2
  Add : Sum
  Add2 : Sum
  Compare To Constant1 : simulink/Logic and Bit Operations/Compare To Constant  relop=>=  const=1  OutDataTypeStr=boolean
  Constant1 : Constant  Value=eps
  Data Type Conversion : DataTypeConversion
  Divide : Product  Inputs=*/
  Gain : Gain  Gain=180/pi
  Math Function : Math  Operator=square  SaturateOnIntegerOverflow=on
  Math Function1 : Math  Operator=square  SaturateOnIntegerOverflow=on
  Product1 : Product  Inputs=3
  Sign : Signum
  Sqrt : Sqrt  AlgorithmType=Newton-Raphson  SaturateOnIntegerOverflow=on
  Trigonometric Function1 : Trigonometry  Operator=atan
  Unary Minus1 : UnaryMinus
  Slip_Angle[deg] : Outport
  wires:
  Gain/1 -> Slip_Angle[deg]/1
  Product1/1 -> Gain/1
  Data Type Conversion/1 -> Product1/2
  Compare To Constant1/1 -> Data Type Conversion/1
  Vy_CoG[m|s]/1 -> Math Function1/1, Divide/1
  Vx_CoG[m|s]/1 -> Sign/1, Math Function/1, Add2/1
  Math Function/1 -> Add/1
  Math Function1/1 -> Add/2
  Add/1 -> Sqrt/1
  Sqrt/1 -> Compare To Constant1/1
  Divide/1 -> Trigonometric Function1/1
  Add2/1 -> Divide/2
  Constant1/1 -> Add2/2
  Trigonometric Function1/1 -> Product1/1
  Sign/1 -> Unary Minus1/1
  Unary Minus1/1 -> Product1/3

== system PC_Simulator_Lib/Drive_Train/4_Wheels_drive_train_and_Brake/RL/Alpha_Kappa_Selector2/alpha_calc/front ==
  Vy : Inport
  Vx : Inport  Port=2
  steering_angle : Inport  Port=3
  Constant : Constant  Value=0.001
  Divide : Product  Inputs=*/
  Fcn : Fcn  Expr=atan(u)
  Gain : Gain  Gain=180/pi
  Relational Operator : RelationalOperator  OutDataTypeStr=boolean
  Subsystem1 : Subsystem
  Subtract : Sum  Inputs=+-
  Switch : Switch  Threshold=1
  alpha : Outport
  wires:
  Relational Operator/1 -> Switch/2
  Constant/1 -> Switch/3, Relational Operator/2
  steering_angle/1 -> Subtract/1
  Subtract/1 -> Gain/1
  Divide/1 -> Fcn/1
  Gain/1 -> alpha/1
  Fcn/1 -> Subtract/2
  Switch/1 -> Divide/2
  Vy/1 -> Subsystem1/1(In1)
  Vx/1 -> Relational Operator/1, Switch/1
  Subsystem1/1(Out1) -> Divide/1

== system PC_Simulator_Lib/Drive_Train/4_Wheels_drive_train_and_Brake/RR/Alpha_Kappa_Selector2/Dynamik Anteil2/Subsystem3 ==
  In1 : Inport
  Abs : Abs  SaturateOnIntegerOverflow=on
  In3_Switch : Constant
  Relational Operator : RelationalOperator
  Switch : Switch  Threshold=1  SaturateOnIntegerOverflow=on
  Out1 : Outport
  wires:
  In1/1 -> Switch/1, Abs/1
  Abs/1 -> Relational Operator/1
  In3_Switch/1 -> Relational Operator/2, Switch/3
  Relational Operator/1 -> Switch/2
  Switch/1 -> Out1/1

== system PC_Simulator_Lib/Drive_Train/4_Wheels_drive_train_and_Brake/RR/Alpha_Kappa_Selector2/alpha_calc/Slip_angle_Calculation_From_Vx_and_Vy1 ==
  Vx_CoG[m|s] : Inport
  Vy_CoG[m|s] : Inport  Port=2
  Add : Sum
  Add2 : Sum
  Compare To Constant1 : simulink/Logic and Bit Operations/Compare To Constant  relop=>=  const=1  OutDataTypeStr=boolean
  Constant1 : Constant  Value=eps
  Data Type Conversion : DataTypeConversion
  Divide : Product  Inputs=*/
  Gain : Gain  Gain=180/pi
  Math Function : Math  Operator=square  SaturateOnIntegerOverflow=on
  Math Function1 : Math  Operator=square  SaturateOnIntegerOverflow=on
  Product1 : Product  Inputs=3
  Sign : Signum
  Sqrt : Sqrt  AlgorithmType=Newton-Raphson  SaturateOnIntegerOverflow=on
  Trigonometric Function1 : Trigonometry  Operator=atan
  Unary Minus1 : UnaryMinus
  Slip_Angle[deg] : Outport
  wires:
  Gain/1 -> Slip_Angle[deg]/1
  Product1/1 -> Gain/1
  Data Type Conversion/1 -> Product1/2
  Compare To Constant1/1 -> Data Type Conversion/1
  Vy_CoG[m|s]/1 -> Math Function1/1, Divide/1
  Vx_CoG[m|s]/1 -> Sign/1, Math Function/1, Add2/1
  Math Function/1 -> Add/1
  Math Function1/1 -> Add/2
  Add/1 -> Sqrt/1
  Sqrt/1 -> Compare To Constant1/1
  Divide/1 -> Trigonometric Function1/1
  Add2/1 -> Divide/2
  Constant1/1 -> Add2/2
  Trigonometric Function1/1 -> Product1/1
  Sign/1 -> Unary Minus1/1
  Unary Minus1/1 -> Product1/3

== system PC_Simulator_Lib/Drive_Train/4_Wheels_drive_train_and_Brake/RR/Alpha_Kappa_Selector2/alpha_calc/front ==
  Vy : Inport
  Vx : Inport  Port=2
  steering_angle : Inport  Port=3
  Constant : Constant  Value=0.001
  Divide : Product  Inputs=*/
  Fcn : Fcn  Expr=atan(u)
  Gain : Gain  Gain=180/pi
  Relational Operator : RelationalOperator  OutDataTypeStr=boolean
  Subsystem1 : Subsystem
  Subtract : Sum  Inputs=+-
  Switch : Switch  Threshold=1
  alpha : Outport
  wires:
  Relational Operator/1 -> Switch/2
  Constant/1 -> Switch/3, Relational Operator/2
  steering_angle/1 -> Subtract/1
  Subtract/1 -> Gain/1
  Divide/1 -> Fcn/1
  Gain/1 -> alpha/1
  Fcn/1 -> Subtract/2
  Switch/1 -> Divide/2
  Vy/1 -> Subsystem1/1(In1)
  Vx/1 -> Relational Operator/1, Switch/1
  Subsystem1/1(Out1) -> Divide/1

== system PC_Simulator_Lib/Drive_Train/4_Wheels_drive_train_and_Brake/FL/Alpha_Kappa_Selector2/alpha_calc/front/Subsystem1 ==
  In1 : Inport
  Abs : Abs
  Constant1 : Constant  Value=0.005
  Constant2 : Constant  Value=0
  Relational Operator1 : RelationalOperator  OutDataTypeStr=boolean
  Switch1 : Switch  Threshold=1
  Out1 : Outport
  wires:
  Abs/1 -> Relational Operator1/1
  Constant2/1 -> Switch1/3
  Constant1/1 -> Relational Operator1/2
  Switch1/1 -> Out1/1
  Relational Operator1/1 -> Switch1/2
  In1/1 -> Abs/1, Switch1/1

== system PC_Simulator_Lib/Drive_Train/4_Wheels_drive_train_and_Brake/FR/Alpha_Kappa_Selector2/alpha_calc/front/Subsystem1 ==
  In1 : Inport
  Abs : Abs
  Constant1 : Constant  Value=0.005
  Constant2 : Constant  Value=0
  Relational Operator1 : RelationalOperator  OutDataTypeStr=boolean
  Switch1 : Switch  Threshold=1
  Out1 : Outport
  wires:
  Abs/1 -> Relational Operator1/1
  Constant2/1 -> Switch1/3
  Constant1/1 -> Relational Operator1/2
  Switch1/1 -> Out1/1
  Relational Operator1/1 -> Switch1/2
  In1/1 -> Abs/1, Switch1/1

== system PC_Simulator_Lib/Drive_Train/4_Wheels_drive_train_and_Brake/RL/Alpha_Kappa_Selector2/alpha_calc/front/Subsystem1 ==
  In1 : Inport
  Abs : Abs
  Constant1 : Constant  Value=0.005
  Constant2 : Constant  Value=0
  Relational Operator1 : RelationalOperator  OutDataTypeStr=boolean
  Switch1 : Switch  Threshold=1
  Out1 : Outport
  wires:
  Abs/1 -> Relational Operator1/1
  Constant2/1 -> Switch1/3
  Constant1/1 -> Relational Operator1/2
  Switch1/1 -> Out1/1
  Relational Operator1/1 -> Switch1/2
  In1/1 -> Abs/1, Switch1/1

== system PC_Simulator_Lib/Drive_Train/4_Wheels_drive_train_and_Brake/RR/Alpha_Kappa_Selector2/alpha_calc/front/Subsystem1 ==
  In1 : Inport
  Abs : Abs
  Constant1 : Constant  Value=0.005
  Constant2 : Constant  Value=0
  Relational Operator1 : RelationalOperator  OutDataTypeStr=boolean
  Switch1 : Switch  Threshold=1
  Out1 : Outport
  wires:
  Abs/1 -> Relational Operator1/1
  Constant2/1 -> Switch1/3
  Constant1/1 -> Relational Operator1/2
  Switch1/1 -> Out1/1
  Relational Operator1/1 -> Switch1/2
  In1/1 -> Abs/1, Switch1/1

== matlab function Drive_Train/4_Wheels_drive_train_and_Brake/FL/Fx_calculator ==
  data: lambda input double; Fx output double; alpha input double; Fz input double; mue input double
 function Fx = FM_Fx(lambda,alpha,Fz,mue)
% This block supports an embeddable subset of the MATLAB language.
% See the help menu for details. 

%% Längstkraft
kappa=lambda;
a=tan(alpha*pi/180);
F_z=Fz;
% Parameter
p_Cx1=1.685;
p_Ex1=0.344;
p_Ex2=0.095;
p_Ex3=-0.02;
p_Ex4=0;
p_Kx1=21.51;
p_Kx2=-0.163;
p_Kx3=0.245;
p_Hx1=0;
p_Hx2=0;
p_Vx1=0;
p_Vx2=0;
r_Cx1=1.0902;
r_Bx1=12.35;
r_Bx2=-10.77;
r_Bx3=0;
r_Ex1=0;
r_Ex2=0;
r_Hx1=0.007;            %r_Hx1=0.007;
gamma=0;
lambda_xa=1;
lambda_Cx=1;
lambda_Ex=1;
lambda_Hx=1;
lambda_Vx=1;
lambda_Kxkappa=1;
% Unter der Annahme, dass die Vertikallast unverändert bleibt:
df_z=0;

%F_z=5500;
%mue=0.7;
chi_1=1;

% Berechnung:

B_xa=(r_Bx1+r_Bx3*gamma^2)*cos(atan(r_Bx2*kappa))*lambda_xa;
C_xa=r_Cx1;
E_xa=r_Ex1+r_Ex2*df_z;

S_Hxa=r_Hx1;
a_S=a+S_Hxa;

G_xa0=cos(C_xa*atan(B_xa*S_Hxa-E_xa*(B_xa*S_Hxa-atan(B_xa*S_Hxa))));
G_xa=cos(C_xa*atan(B_xa*a_S-E_xa*(B_xa*a_S-atan(B_xa*a_S))))/G_xa0;

K_xkappa=F_z*(p_Kx1+p_Kx2*df_z)*exp(p_Kx3*df_z)*lambda_Kxkappa;
C_x=p_Cx1*lambda_Cx;
D_x=mue*F_z*chi_1;
B_x=K_xkappa/(C_x*D_x+eps);
E_x=(p_Ex1+p_Ex2*df_z+p_Ex3*df_z^2)*(1-p_Ex4*sign(kappa))*lambda_Ex;

S_Vx=F_z*(p_Vx1+p_Vx2*df_z)*lambda_Vx*lambda_Hx*chi_1;
S_Hx=(p_Hx1+p_Hx2*df_z)*lambda_Hx;
kappa_x=kappa+S_Hx;

F_x0 = D_x*sin(C_x*atan(B_x*kappa_x-E_x*(B_x*kappa_x-atan(B_x*kappa_x))))+S_Vx;
% F_x0 = D_x*sin(C_x*atan(B_x*kappa_x-E_x.*(B_x*kappa_x-atan(B_x*kappa_x))))+S_Vx;
F_x = G_xa*F_x0;
% if F_x>249;
%     F_x=249;
% end
Fx=F_x;

== stateflow chart Drive_Train/Gearbox/Automatic_Gear_box_Controller ==
  state first
    gear=1;
  state second
    gear=2;
  state third
    gear=3;
  state fourth
    gear=4;
  state neutral
    gear=0;
  state reverse
    gear= 6;
  state fifth
    gear=5;
  second -> third [order 2] : [velocity>30&& omega>4000]
  third -> fourth [order 2] : [velocity>60&& omega>4000]
  (default) -> neutral
  first -> second [order 1] : [velocity>10&& omega>4000]
  fourth -> fifth [order 3] : [velocity>90&& omega>4000]
  reverse -> neutral : [DNR==0]
  neutral -> first [order 1] : [DNR==1]
  second -> neutral [order 3] : [DNR==0]
  second -> first [order 1] : [velocity<5]
  third -> second [order 1] : [velocity<30]
  third -> neutral [order 3] : [DNR==0]
  fourth -> third [order 1] : [velocity<50]
  first -> neutral [order 2] : [DNR==0]
  fourth -> neutral [order 2] : [DNR==0]
  fifth -> fourth [order 1] : [velocity<80]
  fifth -> neutral [order 2] : [DNR==0]
  neutral -> reverse [order 2] : [DNR==-1&& velocity<1]
  data: velocity input double; DNR input double; gear output double; omega input double

== matlab function Drive_Train/4_Wheels_drive_train_and_Brake/FL/Fy_calculator ==
  data: lambda input double; Fy output double; alpha input double; V_x input double; Fz input double; mue input double

function Fy = FM_Fy(lambda,alpha,V_x,Fz,mue)
% This block supports an embeddable subset of the MATLAB language.
% See the help menu for details. 
%% Querkraft

kappa=lambda;
a=tan(alpha*pi/180);
%if V_x >=0 
 %   sign=1;
%else
 %   sign=-1;
%end
a_star=tan(alpha*pi/180)*sign(V_x);
F_z=Fz;
%Parameter

p_Cy1=1.193;
p_Ey1=-1.003;
p_Ey2=-0.532;
p_Ey3=-0.083;
p_Ey4=-4.787;
p_Ey5=0;
p_Ky1=14.95;
p_Ky2=2.13;
p_Ky3=-0.028;
p_Ky4=2;
p_Ky5=0;
p_Ky6=2.5;
p_Ky7=0;
p_Hy1=0;
p_Hy2=0;
p_Vy1=0;
p_Vy2=0;
p_Vy3=0;
p_Vy4=0;
r_By1=6.461;
r_By2=4.196;
r_By3=-0.015;
r_Cy1=1.081;
r_Ey1=0;
r_Ey2=0;
r_Hy1=0;
r_Hy2=0;
r_Vy1=0;
r_Vy2=0;
r_Vy3=0;
r_Vy4=0;
r_Vy5=0;
r_Vy6=0;

lambda_ykappa=1;
lambda_Fz0=1;
lambda_Kya=1;
lambda_Cy=1;
lambda_Vy=1;
lambda_muey=1;
lambda_Hy=1;
lambda_Kygamma=1;
lambda_Ey=1;
lambda_Vykappa=1;

% Unter der Annahme, dass die Vertikallast unverändert bleibt:
df_z=0;

%F_z=5500;
%mue=0.7;
chi_0=1;
chi_1=1;
chi_2=1;
chi_3=1;
chi_4=1;

% Annamhe, dass der Sturz bei null bleibt;

gamma=0;

% Berechnung

B_ykappa=(r_By1+r_By3*gamma^2)*cos(atan(r_By2*(a_star-r_By3)))*lambda_ykappa;
C_ykappa=r_Cy1;
E_ykappa=r_Ey1+r_Ey2*df_z;

S_Hykappa=r_Hy1+r_Hy2*df_z;
kappa_S=kappa+S_Hykappa;

G_ykappa0=cos(C_ykappa*atan(B_ykappa*S_Hykappa-E_ykappa*(B_ykappa*S_Hykappa-atan(B_ykappa*S_Hykappa))));
G_ykappa=cos(C_ykappa*atan(B_ykappa*kappa_S-E_ykappa*(B_ykappa*kappa_S-atan(B_ykappa*kappa_S))))/G_ykappa0;
% G_ykappa=cos(C_ykappa*atan(B_ykappa.*kappa_S-E_ykappa*(B_ykappa.*kappa_S-atan(B_ykappa.*kappa_S))))/G_ykappa0;















K_ygamma0=F_z*(p_Ky6+p_Ky7*df_z)*lambda_Kygamma;
S_Vygamma=F_z*(p_Vy3+p_Vy4*df_z)*gamma*lambda_Kygamma*lambda_muey*chi_2;
K_ya=p_Ky1*lambda_Fz0*F_z*sin(p_Ky4*atan(F_z/((p_Ky2+p_Ky5*gamma^2)*lambda_Fz0*F_z)))/(1+p_Ky3*gamma^2)*chi_3*lambda_Kya;
S_Vy=F_z*(p_Vy1+p_Vy2*df_z)*lambda_Vy*lambda_muey*chi_2+S_Vygamma;
S_Hy=(p_Hy1+p_Hy2*df_z)*lambda_Hy+(K_ygamma0*gamma-S_Vygamma)*chi_0/(K_ya+eps)+chi_4-1;

a_y=a+S_Hy;

D_Vykappa=mue*F_z*(r_Vy1+r_Vy2*df_z+r_Vy3*gamma)*cos(atan(r_Vy4*a))*chi_2;
S_Vykappa=D_Vykappa*sin(r_Vy5*atan(r_Vy6*kappa))*lambda_Vykappa;

C_y=p_Cy1*lambda_Cy;
D_y=mue*F_z*chi_2;
B_y=K_ya/(C_y*D_y+eps);
E_y=(p_Ey1+p_Ey2*df_z)*(1+p_Ey5*gamma^2-(p_Ey3+p_Ey4*gamma)*sign(a_y))*lambda_Ey;

F_y0=D_y*sin(C_y*atan(B_y*a_y-E_y*(B_y*a_y-atan(B_y*a_y))))+S_Vy;

F_y=G_ykappa*F_y0+S_Vykappa;

Fy=F_y;

== matlab function Comunication_with_visualisation_Realtime/Embedded MATLAB Function ==
  data: u input double; y output double
function y = fcn(u)
%#eml

y = typecast(u,'uint8');

== matlab function Drive_Train/4_Wheels_drive_train_and_Brake/RL/Fx_calculator ==
  data: lambda input double; Fx output double; alpha input double; Fz input double; mue input double
 function Fx = FM_Fx(lambda,alpha,Fz,mue)
% This block supports an embeddable subset of the MATLAB language.
% See the help menu for details. 

%% Längstkraft
kappa=lambda;
a=tan(alpha*pi/180);
F_z=Fz;
% Parameter
p_Cx1=1.685;
p_Ex1=0.344;
p_Ex2=0.095;
p_Ex3=-0.02;
p_Ex4=0;
p_Kx1=21.51;
p_Kx2=-0.163;
p_Kx3=0.245;
p_Hx1=0;
p_Hx2=0;
p_Vx1=0;
p_Vx2=0;
r_Cx1=1.0902;
r_Bx1=12.35;
r_Bx2=-10.77;
r_Bx3=0;
r_Ex1=0;
r_Ex2=0;
r_Hx1=0.007;            %r_Hx1=0.007;
gamma=0;
lambda_xa=1;
lambda_Cx=1;
lambda_Ex=1;
lambda_Hx=1;
lambda_Vx=1;
lambda_Kxkappa=1;
% Unter der Annahme, dass die Vertikallast unverändert bleibt:
df_z=0;

%F_z=5500;
%mue=0.7;
chi_1=1;

% Berechnung:

B_xa=(r_Bx1+r_Bx3*gamma^2)*cos(atan(r_Bx2*kappa))*lambda_xa;
C_xa=r_Cx1;
E_xa=r_Ex1+r_Ex2*df_z;

S_Hxa=r_Hx1;
a_S=a+S_Hxa;

G_xa0=cos(C_xa*atan(B_xa*S_Hxa-E_xa*(B_xa*S_Hxa-atan(B_xa*S_Hxa))));
G_xa=cos(C_xa*atan(B_xa*a_S-E_xa*(B_xa*a_S-atan(B_xa*a_S))))/G_xa0;

K_xkappa=F_z*(p_Kx1+p_Kx2*df_z)*exp(p_Kx3*df_z)*lambda_Kxkappa;
C_x=p_Cx1*lambda_Cx;
D_x=mue*F_z*chi_1;
B_x=K_xkappa/(C_x*D_x+eps);
E_x=(p_Ex1+p_Ex2*df_z+p_Ex3*df_z^2)*(1-p_Ex4*sign(kappa))*lambda_Ex;

S_Vx=F_z*(p_Vx1+p_Vx2*df_z)*lambda_Vx*lambda_Hx*chi_1;
S_Hx=(p_Hx1+p_Hx2*df_z)*lambda_Hx;
kappa_x=kappa+S_Hx;

F_x0 = D_x*sin(C_x*atan(B_x*kappa_x-E_x*(B_x*kappa_x-atan(B_x*kappa_x))))+S_Vx;
% F_x0 = D_x*sin(C_x*atan(B_x*kappa_x-E_x.*(B_x*kappa_x-atan(B_x*kappa_x))))+S_Vx;
F_x = G_xa*F_x0;
% if F_x>249;
%     F_x=249;
% end
Fx=F_x;
